simulink model "linearization_sqrt"  (R2023b)
settings: Solver=FixedStepDiscrete  StartTime=0  StopTime=5  FixedStep=1  RelTol=1e-3
undefined symbols (not defined in the file): theta0
settings Model: Creator=alfre  LastModifiedBy=alfre

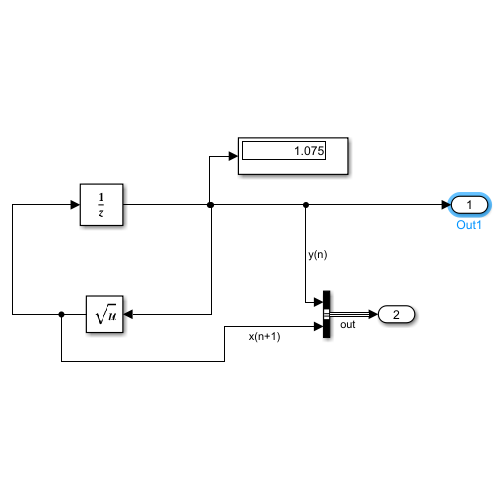
[thumbnail: Simulink's stored preview of the top-level diagram]
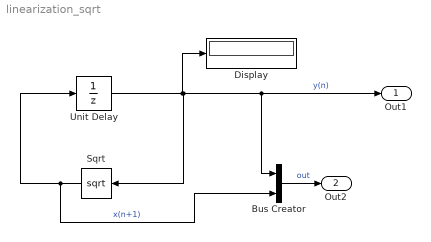
== system linearization_sqrt ==
  Bus Creator : BusCreator  Inputs=2
  Display : Display
  Sqrt : Sqrt
  Unit Delay : UnitDelay  InitialCondition=theta0  SampleTime=-1  HasFrameUpgradeWarning=on
  Out1 : Outport  PortDimensions=2
  Out2 : Outport  Port=2
  wires:
  Unit Delay/1 -> Display/1, Bus Creator/1, Out1/1, Sqrt/1  "y(n)"
  Sqrt/1 -> Bus Creator/2, Unit Delay/1  "x(n+1)"
  Bus Creator/1 -> Out2/1  "out"
